simulink model "stm32f4_target_apds_9301"  (Simulink 7.3)
settings: Solver=FixedStepDiscrete  SolverMode=SingleTasking  StartTime=0.0  StopTime=1  RelTol=1e-3
PreLoadFcn:
  | waijung.modelPreload; % Required for working with Waijung Blockset. Do not remove.
undefined symbols (not defined in the file): HSEOSC, Link, LQFP176, ST, STM32F417IG
libraries: simulink x19, stm32f4_device_config_lib x1
(part 2 of 2)

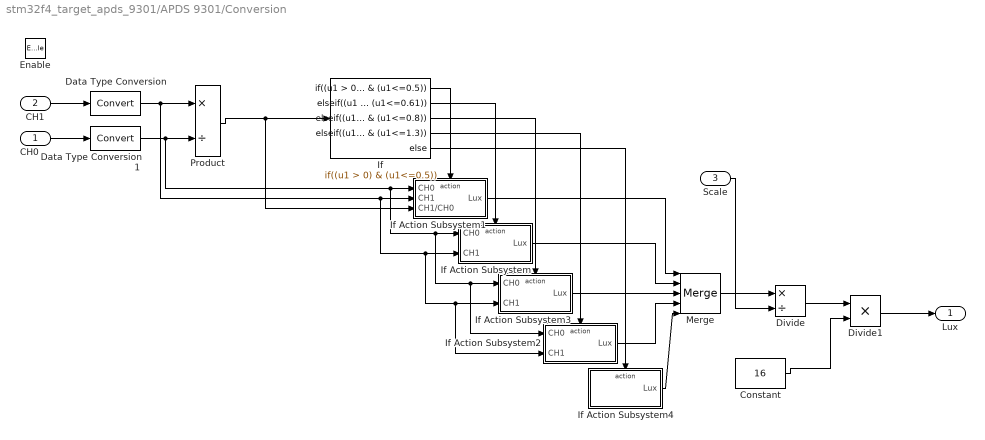
== system stm32f4_target_apds_9301/APDS 9301/Conversion ==
  CH0 : Inport  OutDataType=fixdt(1, 16)  OutScaling=2^0
  CH1 : Inport  Port=2  OutDataType=fixdt(1, 16)  OutScaling=2^0
  Scale : Inport  Port=3  OutDataType=fixdt(1, 16)  OutScaling=2^0
  Enable : EnablePort
  Constant : Constant  Value=16  OutDataType=fixdt(1, 16)  OutScaling=2^0
  Data Type Conversion : DataTypeConversion  OutDataType=fixdt(1, 16)  OutScaling=2^0
  Data Type Conversion1 : DataTypeConversion  OutDataType=fixdt(1, 16)  OutScaling=2^0
  Divide : Product  Inputs=*/  OutDataType=fixdt(1, 16)  OutScaling=2^-10
  Divide1 : Product  Inputs=**  OutDataType=fixdt(1, 16)  OutScaling=2^-10
  If : If  IfExpression=(u1 > 0) & (u1<=0.5)  ElseIfExpressions=(u1 > 0.5) & (u1<=0.61),(u1 > 0.61) & (u1<=0.8),(u1 > 0.8) & (u1<=1.3)
  If Action Subsystem : Subsystem  TreatAsAtomicUnit=on
  If Action Subsystem1 : Subsystem  TreatAsAtomicUnit=on
  If Action Subsystem2 : Subsystem  TreatAsAtomicUnit=on
  If Action Subsystem3 : Subsystem  TreatAsAtomicUnit=on
  If Action Subsystem4 : Subsystem  TreatAsAtomicUnit=on
  Merge : Merge  Inputs=5
  Product : Product  Inputs=*/  OutDataType=fixdt(1, 16)  OutScaling=2^0  RndMeth=Zero
  Lux : Outport  OutDataType=fixdt(1, 16)  OutScaling=2^0
  wires:
  Merge/1 -> Divide/1
  If Action Subsystem4/1(Lux) -> Merge/5
  If Action Subsystem2/1(Lux) -> Merge/4
  If Action Subsystem3/1(Lux) -> Merge/3
  If Action Subsystem/1(Lux) -> Merge/2
  If Action Subsystem1/1(Lux) -> Merge/1
  Divide1/1 -> Lux/1
  Constant/1 -> Divide1/2
  Divide/1 -> Divide1/1
  Scale/1 -> Divide/2
  Data Type Conversion1/1 -> If Action Subsystem2/1(CH0), If Action Subsystem3/1(CH0), If Action Subsystem/1(CH0), If Action Subsystem1/1(CH0), Product/2
  Data Type Conversion/1 -> If Action Subsystem2/2(CH1), If Action Subsystem3/2(CH1), If Action Subsystem/2(CH1), If Action Subsystem1/2(CH1), Product/1
  If/5 -> If Action Subsystem4/Action
  If/4 -> If Action Subsystem2/Action
  If/3 -> If Action Subsystem3/Action
  If/2 -> If Action Subsystem/Action
  If/1 -> If Action Subsystem1/Action
  Product/1 -> If Action Subsystem1/3(CH1/CH0), If/1
  CH0/1 -> Data Type Conversion1/1
  CH1/1 -> Data Type Conversion/1

== system stm32f4_target_apds_9301/APDS 9301/SCALE ==
  note: # Priority: 0
  SlvAddr : Inport
  Constant : Constant  Value=hex2dec('02')  OutDataTypeMode=uint8  OutDataType=fixdt(1, 16)  OutScaling=2^0  OutDataTypeStr=uint8
  Subsystem : Subsystem
  Subsystem1 : Subsystem
  Terminator : Terminator
  Scale : Outport  OutDataType=fixdt(1, 16)  OutScaling=2^0
  wires:
  Constant/1 -> Subsystem/2(Value)
  Subsystem1/1(Conf_scale) -> Scale/1
  Subsystem/1(READY) -> Terminator/1
  SlvAddr/1 -> Subsystem1/1(SlvAddr), Subsystem/1(SlvAddr)

== system stm32f4_target_apds_9301/APDS 9301/APDS_9301_Initialize/Enabled Subsystem ==
  SlvAddr : Inport  OutDataType=fixdt(1, 16)  OutScaling=2^0
  Cmd : Inport  Port=2  OutDataType=fixdt(1, 16)  OutScaling=2^0
  Enable : EnablePort
  I2C Master Read/Write : S-Function  FunctionName=stm32f4_i2c  Parameters=configuration,module,transfer,clkspeed,timeout,sdapin,sclpin,writecount,readcount,inputtypearray,outputtypearray,confstr,sampletime,sampletimestr,blockid  EnableBusSupport=off  mask(stm32f4_i2c){configuration=Transaction, module=1, lastmodule=3, transfer=Blocking, dutycycle=TLow/THigh = 2, clkspeed=400, timeout=25, writecount=2, readcount=0, sdapin=C9, sclpin=A8, waitwritetime=0, inputtypearray=[3 3 3 3], outputtypearray=[1 3], confstr=["C","9","A","8","1","1","6","0","I2C_DutyCycle_2","0","off"], sampletime=-1, sampletimestr=0.5, blockid=APDS9301APDS_9301_InitializeEnabledSubsystemI2CMasterReadWrite}
      mask prompts: module "I2C Module"; lastmodule "Last module"; transfer "Transfer mode"; dutycycle "Duty cycle in fast mode"; clkspeed "Clock speed (kHz)"; timeout "Timeout (ms)"; writecount "Bytes write count"; readcount "Bytes read count"; sdapin "SDA pin"; sclpin "SCL pin"; waitwritetime "Wait write time (ms), default is 0"; inputtypearray "Input type array"; outputtypearray "Output type array"; confstr "Configuration string"; sampletime "Sample time (sec)"; sampletimestr "Compiled sample time (sec) in string"
      mask init:
      | stm32f4_i2c_callback('init');
      mask Help: web(fullfile(waijungdocroot,'stm32f4_i2c_readwrite.htm'), '-browser')
      mask StyleString: popup(Setup|Transaction),popup(1|2|3),edit,popup(Blocking|Non-blocking),popup(TLow/THigh = 16/9|TLow/THigh = 2),edit,edit,edit,edit,popup(-|C9),popup(-|A8),edit,edit,edit,edit,edit,edit,edit
      mask CallbackString: stm32f4_i2c_callback('configuration');|stm32f4_i2c_callback('module');|||stm32f4_i2c_callback('dutycycle');|||stm32f4_i2c_callback('writecount');|stm32f4_i2c_callback('readcount');|stm32f4_i2c_callback('sdapin');|stm32f4_i2c_callback('sclpin');||||stm32f4_i2c_callback('confstr');|stm32f4_i2c_callback('sampletime');|stm32f4_i2c_callback('sampletimestr');|stm32f4_i2c_callback('blockid');
      mask Display: text(0.5, 0.5, 'Module: I2C1\nTransfer: Blocking\nWrite: 2 bytes\nRead: 0 bytes\nTs (sec): 0.5','ver','middle','hor','center');port_label('input', 1,'SlvAddr');port_label('input', 2,'Wr0 (uint8)');port_label('input', 3,'Wr1 (uint8)');port_label('output', 1,'Status');
  Power ON : Constant  Value=3  OutDataTypeMode=uint8  OutDataType=fixdt(1, 16)  OutScaling=2^0  OutDataTypeStr=uint8
  Terminator : Terminator
  wires:
  I2C Master Read/Write/1 -> Terminator/1
  Power ON/1 -> I2C Master Read/Write/3
  Cmd/1 -> I2C Master Read/Write/2
  SlvAddr/1 -> I2C Master Read/Write/1

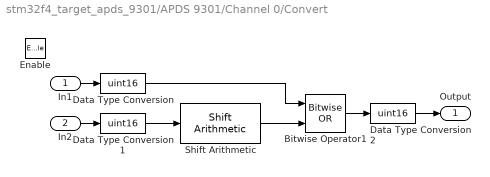
== system stm32f4_target_apds_9301/APDS 9301/Channel 0/Convert ==
  In1 : Inport
  In2 : Inport  Port=2
  Enable : EnablePort
  Bitwise Operator1 : simulink/Logic and Bit Operations/Bitwise Operator  logicop=OR  UseBitMask=off  NumInputPorts=2  BitMask=bin2dec('11011001')  BitMaskRealWorld=Stored Integer
  Data Type Conversion : DataTypeConversion  OutDataTypeMode=uint16  OutDataType=fixdt(1, 16)  OutScaling=2^0  OutDataTypeStr=uint16
  Data Type Conversion1 : DataTypeConversion  OutDataTypeMode=uint16  OutDataType=fixdt(1, 16)  OutScaling=2^0  OutDataTypeStr=uint16
  Data Type Conversion2 : DataTypeConversion  OutDataTypeMode=uint16  OutDataType=fixdt(1, 16)  OutScaling=2^0  OutDataTypeStr=uint16
  Shift Arithmetic : simulink/Logic and Bit Operations/Shift Arithmetic  SystemSampleTime=-1  nBitShiftRight=-8  nBinPtShiftRight=0
  Output : Outport
  wires:
  Data Type Conversion/1 -> Bitwise Operator1/1
  Data Type Conversion1/1 -> Shift Arithmetic/1
  In2/1 -> Data Type Conversion1/1
  Data Type Conversion2/1 -> Output/1
  In1/1 -> Data Type Conversion/1
  Bitwise Operator1/1 -> Data Type Conversion2/1
  Shift Arithmetic/1 -> Bitwise Operator1/2

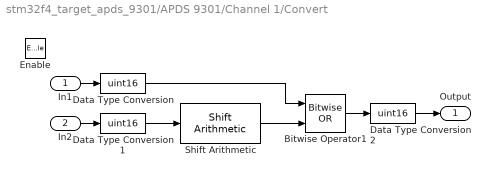
== system stm32f4_target_apds_9301/APDS 9301/Channel 1/Convert ==
  In1 : Inport
  In2 : Inport  Port=2
  Enable : EnablePort
  Bitwise Operator1 : simulink/Logic and Bit Operations/Bitwise Operator  logicop=OR  UseBitMask=off  NumInputPorts=2  BitMask=bin2dec('11011001')  BitMaskRealWorld=Stored Integer
  Data Type Conversion : DataTypeConversion  OutDataTypeMode=uint16  OutDataType=fixdt(1, 16)  OutScaling=2^0  OutDataTypeStr=uint16
  Data Type Conversion1 : DataTypeConversion  OutDataTypeMode=uint16  OutDataType=fixdt(1, 16)  OutScaling=2^0  OutDataTypeStr=uint16
  Data Type Conversion2 : DataTypeConversion  OutDataTypeMode=uint16  OutDataType=fixdt(1, 16)  OutScaling=2^0  OutDataTypeStr=uint16
  Shift Arithmetic : simulink/Logic and Bit Operations/Shift Arithmetic  SystemSampleTime=-1  nBitShiftRight=-8  nBinPtShiftRight=0
  Output : Outport
  wires:
  Shift Arithmetic/1 -> Bitwise Operator1/2
  Bitwise Operator1/1 -> Data Type Conversion2/1
  In1/1 -> Data Type Conversion/1
  Data Type Conversion2/1 -> Output/1
  In2/1 -> Data Type Conversion1/1
  Data Type Conversion1/1 -> Shift Arithmetic/1
  Data Type Conversion/1 -> Bitwise Operator1/1

== system stm32f4_target_apds_9301/APDS 9301/Conversion/If Action Subsystem ==
  CH0 : Inport  OutDataType=fixdt(1, 16)  OutScaling=2^0
  CH1 : Inport  Port=2  OutDataType=fixdt(1, 16)  OutScaling=2^0
  Action Port : ActionPort  ActionType=elseif
  Gain : Gain  Gain=0.0224  ParameterDataType=fixdt(1, 16)  ParameterScaling=2^0  OutDataType=fixdt(1, 16)  OutScaling=2^0
  Gain1 : Gain  Gain=0.031  ParameterDataType=fixdt(1, 16)  ParameterScaling=2^0  OutDataType=fixdt(1, 16)  OutScaling=2^0
  Subtract : Sum  Inputs=+-  OutDataType=fixdt(1, 16)  OutScaling=2^-10
  Lux : Outport  OutDataType=fixdt(1, 16)  OutScaling=2^0
  wires:
  Gain1/1 -> Subtract/2
  Gain/1 -> Subtract/1
  CH1/1 -> Gain1/1
  Subtract/1 -> Lux/1
  CH0/1 -> Gain/1

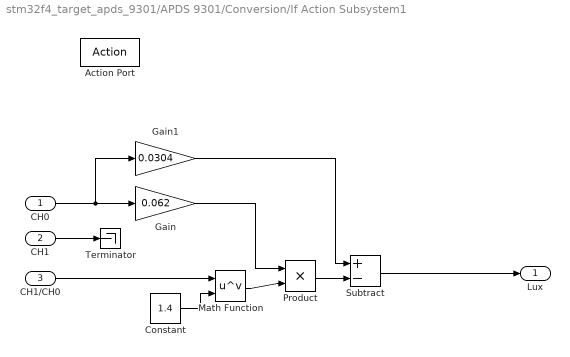
== system stm32f4_target_apds_9301/APDS 9301/Conversion/If Action Subsystem1 ==
  CH0 : Inport  OutDataType=fixdt(1, 16)  OutScaling=2^0
  CH1 : Inport  Port=2  OutDataType=fixdt(1, 16)  OutScaling=2^0
  CH1/CH0 : Inport  Port=3  OutDataType=fixdt(1, 16)  OutScaling=2^0
  Action Port : ActionPort  ActionType=then
  Constant : Constant  Value=1.4  OutDataType=fixdt(1, 16)  OutScaling=2^0
  Gain : Gain  Gain=0.062  ParameterDataType=fixdt(1, 16)  ParameterScaling=2^0  OutDataType=fixdt(1, 16)  OutScaling=2^0
  Gain1 : Gain  Gain=0.0304  ParameterDataType=fixdt(1, 16)  ParameterScaling=2^0  OutDataType=fixdt(1, 16)  OutScaling=2^0
  Math Function : Math  Operator=pow  OutDataType=fixdt(1, 16)  OutScaling=2^0  SaturateOnIntegerOverflow=on
  Product : Product  OutDataType=fixdt(1, 16)  OutScaling=2^0  RndMeth=Zero
  Subtract : Sum  Inputs=+-  OutDataType=fixdt(1, 16)  OutScaling=2^-10
  Terminator : Terminator
  Lux : Outport  OutDataType=fixdt(1, 16)  OutScaling=2^0
  wires:
  CH1/1 -> Terminator/1
  Subtract/1 -> Lux/1
  Product/1 -> Subtract/2
  Gain1/1 -> Subtract/1
  Math Function/1 -> Product/2
  Gain/1 -> Product/1
  CH1/CH0/1 -> Math Function/1
  Constant/1 -> Math Function/2
  CH0/1 -> Gain1/1, Gain/1

== system stm32f4_target_apds_9301/APDS 9301/Conversion/If Action Subsystem2 ==
  CH0 : Inport  OutDataType=fixdt(1, 16)  OutScaling=2^0
  CH1 : Inport  Port=2  OutDataType=fixdt(1, 16)  OutScaling=2^0
  Action Port : ActionPort  ActionType=elseif
  Gain : Gain  Gain=0.00146  ParameterDataType=fixdt(1, 16)  ParameterScaling=2^0  OutDataType=fixdt(1, 16)  OutScaling=2^0
  Gain1 : Gain  Gain=0.00112  ParameterDataType=fixdt(1, 16)  ParameterScaling=2^0  OutDataType=fixdt(1, 16)  OutScaling=2^0
  Subtract : Sum  Inputs=+-  OutDataType=fixdt(1, 16)  OutScaling=2^-10
  Lux : Outport  OutDataType=fixdt(1, 16)  OutScaling=2^0
  wires:
  Gain1/1 -> Subtract/2
  Gain/1 -> Subtract/1
  CH1/1 -> Gain1/1
  Subtract/1 -> Lux/1
  CH0/1 -> Gain/1

== system stm32f4_target_apds_9301/APDS 9301/Conversion/If Action Subsystem3 ==
  CH0 : Inport  OutDataType=fixdt(1, 16)  OutScaling=2^0
  CH1 : Inport  Port=2  OutDataType=fixdt(1, 16)  OutScaling=2^0
  Action Port : ActionPort  ActionType=elseif
  Gain : Gain  Gain=0.0128  ParameterDataType=fixdt(1, 16)  ParameterScaling=2^0  OutDataType=fixdt(1, 16)  OutScaling=2^0
  Gain1 : Gain  Gain=0.0153  ParameterDataType=fixdt(1, 16)  ParameterScaling=2^0  OutDataType=fixdt(1, 16)  OutScaling=2^0
  Subtract : Sum  Inputs=+-  OutDataType=fixdt(1, 16)  OutScaling=2^-10
  Lux : Outport  OutDataType=fixdt(1, 16)  OutScaling=2^0
  wires:
  Gain1/1 -> Subtract/2
  Gain/1 -> Subtract/1
  CH1/1 -> Gain1/1
  Subtract/1 -> Lux/1
  CH0/1 -> Gain/1

== system stm32f4_target_apds_9301/APDS 9301/Conversion/If Action Subsystem4 ==
  Action Port : ActionPort  ActionType=else
  Constant : Constant  Value=0  OutDataType=fixdt(1, 16)  OutScaling=2^0
  Lux : Outport  OutDataType=fixdt(1, 16)  OutScaling=2^0
  wires:
  Constant/1 -> Lux/1

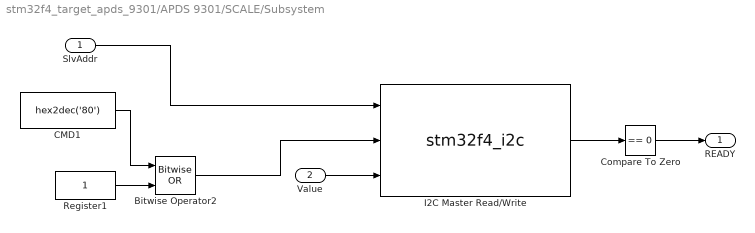
== system stm32f4_target_apds_9301/APDS 9301/SCALE/Subsystem ==
  SlvAddr : Inport
  Value : Inport  Port=2
  Bitwise Operator2 : simulink/Logic and Bit Operations/Bitwise Operator  logicop=OR  UseBitMask=off  NumInputPorts=2  BitMask=bin2dec('11011001')  BitMaskRealWorld=Stored Integer
  CMD1 : Constant  Value=hex2dec('80')  OutDataTypeMode=uint8  OutDataType=fixdt(1, 16)  OutScaling=2^0  OutDataTypeStr=uint8
  Compare To Zero : simulink/Logic and Bit Operations/Compare To Zero  SystemSampleTime=-1  relop===  LogicOutDataTypeMode=uint8  ZeroCross=off
  I2C Master Read/Write : S-Function  FunctionName=stm32f4_i2c  Parameters=configuration,module,transfer,clkspeed,timeout,sdapin,sclpin,writecount,readcount,inputtypearray,outputtypearray,confstr,sampletime,sampletimestr,blockid  EnableBusSupport=off  mask(stm32f4_i2c){configuration=Transaction, module=1, lastmodule=3, transfer=Blocking, dutycycle=TLow/THigh = 2, clkspeed=400, timeout=25, writecount=2, readcount=0, sdapin=C9, sclpin=A8, waitwritetime=0, inputtypearray=[3 3 3 3], outputtypearray=[1 3], confstr=["C","9","A","8","1","1","6","0","I2C_DutyCycle_2","0","off"], sampletime=-1, sampletimestr=0.5, blockid=APDS9301SCALESubsystemI2CMasterReadWrite}
      mask prompts: module "I2C Module"; lastmodule "Last module"; transfer "Transfer mode"; dutycycle "Duty cycle in fast mode"; clkspeed "Clock speed (kHz)"; timeout "Timeout (ms)"; writecount "Bytes write count"; readcount "Bytes read count"; sdapin "SDA pin"; sclpin "SCL pin"; waitwritetime "Wait write time (ms), default is 0"; inputtypearray "Input type array"; outputtypearray "Output type array"; confstr "Configuration string"; sampletime "Sample time (sec)"; sampletimestr "Compiled sample time (sec) in string"
      mask init:
      | stm32f4_i2c_callback('init');
      mask Help: web(fullfile(waijungdocroot,'stm32f4_i2c_readwrite.htm'), '-browser')
      mask StyleString: popup(Setup|Transaction),popup(1|2|3),edit,popup(Blocking|Non-blocking),popup(TLow/THigh = 16/9|TLow/THigh = 2),edit,edit,edit,edit,popup(-|C9),popup(-|A8),edit,edit,edit,edit,edit,edit,edit
      mask CallbackString: stm32f4_i2c_callback('configuration');|stm32f4_i2c_callback('module');|||stm32f4_i2c_callback('dutycycle');|||stm32f4_i2c_callback('writecount');|stm32f4_i2c_callback('readcount');|stm32f4_i2c_callback('sdapin');|stm32f4_i2c_callback('sclpin');||||stm32f4_i2c_callback('confstr');|stm32f4_i2c_callback('sampletime');|stm32f4_i2c_callback('sampletimestr');|stm32f4_i2c_callback('blockid');
      mask Display: text(0.5, 0.5, 'Module: I2C1\nTransfer: Blocking\nWrite: 2 bytes\nRead: 0 bytes\nTs (sec): 0.5','ver','middle','hor','center');port_label('input', 1,'SlvAddr');port_label('input', 2,'Wr0 (uint8)');port_label('input', 3,'Wr1 (uint8)');port_label('output', 1,'Status');
  Register1 : Constant  OutDataTypeMode=uint8  OutDataType=fixdt(1, 16)  OutScaling=2^0  OutDataTypeStr=uint8
  READY : Outport  OutDataType=fixdt(1, 16)  OutScaling=2^0
  wires:
  Compare To Zero/1 -> READY/1
  I2C Master Read/Write/1 -> Compare To Zero/1
  Bitwise Operator2/1 -> I2C Master Read/Write/2
  Register1/1 -> Bitwise Operator2/2
  CMD1/1 -> Bitwise Operator2/1
  Value/1 -> I2C Master Read/Write/3
  SlvAddr/1 -> I2C Master Read/Write/1

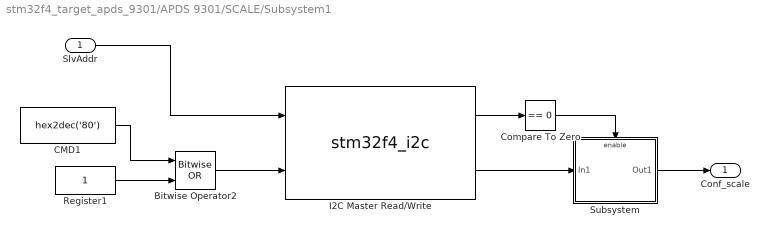
== system stm32f4_target_apds_9301/APDS 9301/SCALE/Subsystem1 ==
  SlvAddr : Inport
  Bitwise Operator2 : simulink/Logic and Bit Operations/Bitwise Operator  logicop=OR  UseBitMask=off  NumInputPorts=2  BitMask=bin2dec('11011001')  BitMaskRealWorld=Stored Integer
  CMD1 : Constant  Value=hex2dec('80')  OutDataTypeMode=uint8  OutDataType=fixdt(1, 16)  OutScaling=2^0  OutDataTypeStr=uint8
  Compare To Zero : simulink/Logic and Bit Operations/Compare To Zero  SystemSampleTime=-1  relop===  LogicOutDataTypeMode=uint8  ZeroCross=off
  I2C Master Read/Write : S-Function  Priority=0  FunctionName=stm32f4_i2c  Parameters=configuration,module,transfer,clkspeed,timeout,sdapin,sclpin,writecount,readcount,inputtypearray,outputtypearray,confstr,sampletime,sampletimestr,blockid  EnableBusSupport=off  mask(stm32f4_i2c){configuration=Transaction, module=1, lastmodule=3, transfer=Blocking, dutycycle=TLow/THigh = 2, clkspeed=400, timeout=25, writecount=1, readcount=1, sdapin=C9, sclpin=A8, waitwritetime=0, inputtypearray=[2 3 3], outputtypearray=[2 3 3], confstr=["C","9","A","8","1","1","6","0","I2C_DutyCycle_2","0","off"], sampletime=-1, sampletimestr=0.5, blockid=APDS9301SCALESubsystem1I2CMasterReadWrite}
      mask prompts: module "I2C Module"; lastmodule "Last module"; transfer "Transfer mode"; dutycycle "Duty cycle in fast mode"; clkspeed "Clock speed (kHz)"; timeout "Timeout (ms)"; writecount "Bytes write count"; readcount "Bytes read count"; sdapin "SDA pin"; sclpin "SCL pin"; waitwritetime "Wait write time (ms), default is 0"; inputtypearray "Input type array"; outputtypearray "Output type array"; confstr "Configuration string"; sampletime "Sample time (sec)"; sampletimestr "Compiled sample time (sec) in string"
      mask init:
      | stm32f4_i2c_callback('init');
      mask Help: web(fullfile(waijungdocroot,'stm32f4_i2c_readwrite.htm'), '-browser')
      mask StyleString: popup(Setup|Transaction),popup(1|2|3),edit,popup(Blocking|Non-blocking),popup(TLow/THigh = 16/9|TLow/THigh = 2),edit,edit,edit,edit,popup(-|C9),popup(-|A8),edit,edit,edit,edit,edit,edit,edit
      mask CallbackString: stm32f4_i2c_callback('configuration');|stm32f4_i2c_callback('module');|||stm32f4_i2c_callback('dutycycle');|||stm32f4_i2c_callback('writecount');|stm32f4_i2c_callback('readcount');|stm32f4_i2c_callback('sdapin');|stm32f4_i2c_callback('sclpin');||||stm32f4_i2c_callback('confstr');|stm32f4_i2c_callback('sampletime');|stm32f4_i2c_callback('sampletimestr');|stm32f4_i2c_callback('blockid');
      mask Display: text(0.5, 0.5, 'Module: I2C1\nTransfer: Blocking\nWrite: 1 bytes\nRead: 1 bytes\nTs (sec): 0.5','ver','middle','hor','center');port_label('input', 1,'SlvAddr');port_label('input', 2,'Wr0 (uint8)');port_label('output', 1,'Status');port_label('output', 2,'Rd0 (uint8)');
  Register1 : Constant  OutDataTypeMode=uint8  OutDataType=fixdt(1, 16)  OutScaling=2^0  OutDataTypeStr=uint8
  Subsystem : Subsystem
  Conf_scale : Outport  OutDataType=fixdt(1, 16)  OutScaling=2^0
  wires:
  Subsystem/1(Out1) -> Conf_scale/1
  I2C Master Read/Write/2 -> Subsystem/1(In1)
  SlvAddr/1 -> I2C Master Read/Write/1
  CMD1/1 -> Bitwise Operator2/1
  Register1/1 -> Bitwise Operator2/2
  Bitwise Operator2/1 -> I2C Master Read/Write/2
  I2C Master Read/Write/1 -> Compare To Zero/1
  Compare To Zero/1 -> Subsystem/Enable

== system stm32f4_target_apds_9301/APDS 9301/SCALE/Subsystem1/Subsystem ==
  In1 : Inport
  Enable : EnablePort
  Bitwise Operator : simulink/Logic and Bit Operations/Bitwise Operator  logicop=AND  UseBitMask=on  BitMask=3  BitMaskRealWorld=Stored Integer
  Constant1 : Constant  OutDataType=fixdt(1, 16)  OutScaling=2^0
  Constant2 : Constant  Value=0.034  OutDataType=fixdt(1, 16)  OutScaling=2^0
  Constant3 : Constant  Value=0.252  OutDataType=fixdt(1, 16)  OutScaling=2^0
  Multiport Switch : MultiPortSwitch  Inputs=4  zeroidx=on  OutDataType=fixdt(1, 16)  OutScaling=2^0
  Out1 : Outport
  wires:
  Multiport Switch/1 -> Out1/1
  Constant1/1 -> Multiport Switch/5, Multiport Switch/4
  Constant3/1 -> Multiport Switch/3
  Constant2/1 -> Multiport Switch/2
  In1/1 -> Bitwise Operator/1
  Bitwise Operator/1 -> Multiport Switch/1
